simulink model "cruise_control_model"  (R2020b)
settings: Solver=VariableStepAuto  StartTime=0.0  StopTime=100  RelTol=1e-3
undefined symbols (not defined in the file or in its folder): b, Kd, Ki, Kp, m
settings Model: DataDictionary=datadic3.sldd  Creator=ARPITA  LastModifiedBy=ARPITA
settings DataIOCC: SaveOutput=off  SaveTime=off

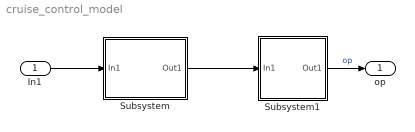
== system cruise_control_model ==
  In1 : Inport  OutDataTypeStr=double  PortDimensions=1  SampleTime=0
  Subsystem : Subsystem
  Subsystem1 : Subsystem
  op : Outport  OutDataTypeStr=double  PortDimensions=1  SampleTime=0
  wires:
  Subsystem/1(Out1) -> Subsystem1/1(In1)
  In1/1 -> Subsystem/1(In1)
  Subsystem1/1(Out1) -> op/1  "op"

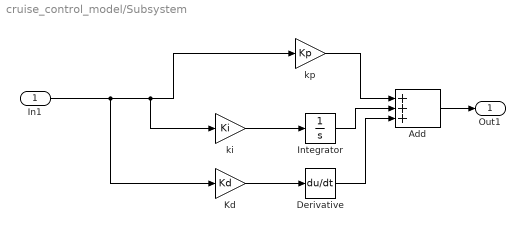
== system cruise_control_model/Subsystem ==
  In1 : Inport
  Add : Sum  Inputs=+++
  Derivative : Derivative
  Integrator : Integrator
  Kd : Gain  Gain=Kd
  ki : Gain  Gain=Ki
  kp : Gain  Gain=Kp
  Out1 : Outport
  wires:
  kp/1 -> Add/1
  ki/1 -> Integrator/1
  Kd/1 -> Derivative/1
  Integrator/1 -> Add/2
  In1/1 -> kp/1, ki/1, Kd/1
  Add/1 -> Out1/1
  Derivative/1 -> Add/3

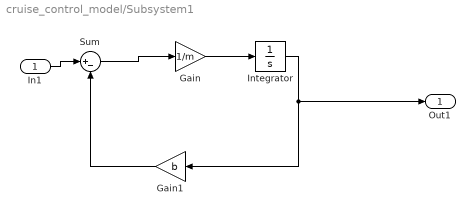
== system cruise_control_model/Subsystem1 ==
  In1 : Inport
  Gain : Gain  Gain=1/m
  Gain1 : Gain  Gain=b
  Integrator : Integrator
  Sum : Sum  Inputs=|+-
  Out1 : Outport
  wires:
  Integrator/1 -> Gain1/1, Out1/1
  Gain1/1 -> Sum/2
  Sum/1 -> Gain/1
  Gain/1 -> Integrator/1
  In1/1 -> Sum/1
